simulink model "RC_circuit"  (R2023a)
settings: Solver=FixedStepAuto  StartTime=0.0  StopTime=10  FixedStep=1e-3
values from neighbouring files (symbols this model uses):
  C = 0.000001    (= 1e-06)    [RC_circuit.m]
  R = 1000    [RC_circuit.m]
settings Model: Creator=Mass  LastModifiedBy=Mass

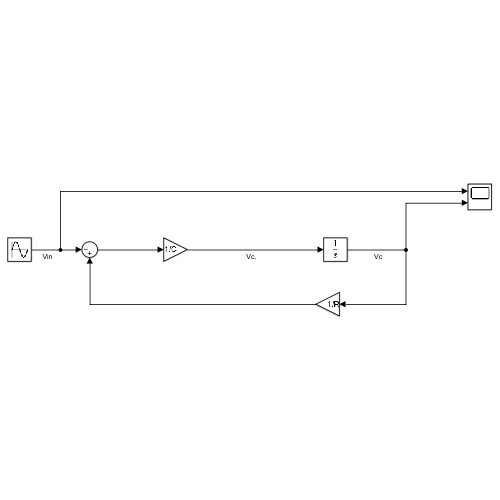
[thumbnail: Simulink's stored preview of the top-level diagram]
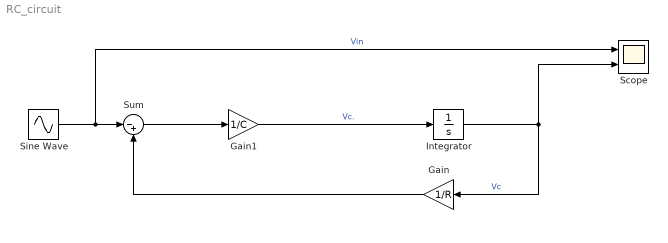
== system RC_circuit ==
  Gain : Gain  Gain=1/R
  Gain1 : Gain  Gain=1/C
  Integrator : Integrator  InitialCondition=0.01
  Scope : Scope  NumInputPorts=2
  Sine Wave : Sin  Amplitude=5  Frequency=2*pi  SampleTime=0
  Sum : Sum  Inputs=|-+
  wires:
  Sum/1 -> Gain1/1
  Gain1/1 -> Integrator/1  "Vc."
  Sine Wave/1 -> Scope/1, Sum/1  "Vin"
  Integrator/1 -> Scope/2, Gain/1  "Vc"
  Gain/1 -> Sum/2
